simulink model "PenduloCarro2"  (R2017b)
settings: Solver=ode4  StartTime=0.0  StopTime=10.0  FixedStep=0.001  RelTol=1e-3
values from neighbouring files (symbols this model uses):
  g = 9.81    [PenduloInvertido.m]
  l = 0.5    [PenduloInvertido.m]
  m = 0.1    [PenduloInvertido.m]
undefined symbols (not defined in the file or in its folder): K, m1
settings Model: Creator=Benjamin Nicolas  LastModifiedBy=Benjamin Nicolas

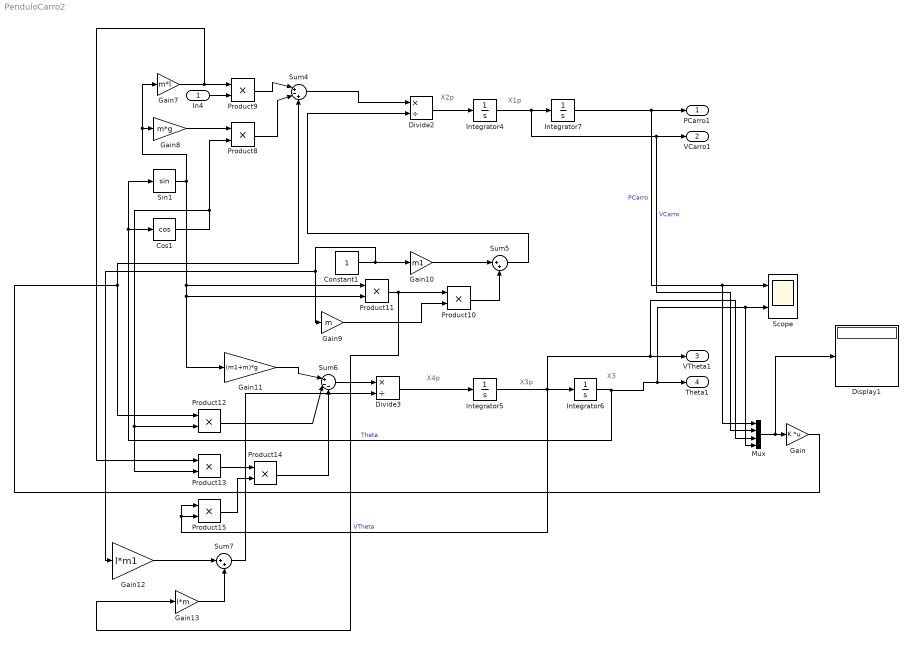
== system PenduloCarro2 ==
  note: X3
  note: X1p
  note: X2p
  note: X4p
  note: X3p
  In4 : Inport
  Constant1 : Constant
  Cos1 : Trigonometry  Operator=cos
  Display1 : Display
  Divide2 : Product  Inputs=*/
  Divide3 : Product  Inputs=*/
  Gain : Gain  Gain=K  Multiplication=Matrix(K*u)
  Gain10 : Gain  Gain=m1
  Gain11 : Gain  Gain=(m1+m)*g
  Gain12 : Gain  Gain=l*m1
  Gain13 : Gain  Gain=l*m
  Gain7 : Gain  Gain=m*l
  Gain8 : Gain  Gain=m*g
  Gain9 : Gain  Gain=m
  Integrator4 : Integrator
  Integrator5 : Integrator  InitialCondition=0.13
  Integrator6 : Integrator
  Integrator7 : Integrator
  Mux : Mux
  Product{8..15} (8 alike) : Product
  Scope : Scope  NumInputPorts=2
  Sin1 : Trigonometry
  Sum4 : Sum  Inputs=|+-+
  Sum5 : Sum  Inputs=|++
  Sum6 : Sum  Inputs=|+--
  Sum7 : Sum  Inputs=|++
  PCarro1 : Outport
  VCarro1 : Outport  Port=2
  VTheta1 : Outport  Port=3
  Theta1 : Outport  Port=4
  wires:
  Gain/1 -> Sum4/3, Product12/1
  Integrator7/1 -> Mux/1, Scope/1, PCarro1/1  "PCarro"
  Product8/1 -> Sum4/2
  Integrator4/1 -> Mux/2, VCarro1/1, Integrator7/1  "VCarro"
  Gain8/1 -> Product8/1
  Gain7/1 -> Product13/1, Product9/1
  Sum7/1 -> Divide3/2
  Product13/1 -> Product14/1
  Sum6/1 -> Divide3/1
  Gain10/1 -> Sum5/1
  Gain12/1 -> Sum7/1
  Gain13/1 -> Sum7/2
  Sum5/1 -> Divide2/2
  Gain11/1 -> Sum6/1
  Gain9/1 -> Product10/2
  Product14/1 -> Sum6/3
  Product9/1 -> Sum4/1
  In4/1 -> Product9/2
  Product12/1 -> Sum6/2
  Sin1/1 -> Gain11/1, Product11/2, Product11/1, Gain7/1, Gain8/1
  Cos1/1 -> Product12/2, Product13/2, Product8/2
  Product10/1 -> Sum5/2
  Constant1/1 -> Gain12/1, Gain9/1, Gain10/1
  Integrator5/1 -> Mux/3, VTheta1/1, Integrator6/1, Product15/2, Product15/1  "VTheta"
  Product15/1 -> Product14/2
  Integrator6/1 -> Mux/4, Scope/2, Theta1/1, Sin1/1, Cos1/1  "Theta"
  Product11/1 -> Gain13/1, Product10/1
  Sum4/1 -> Divide2/1
  Divide3/1 -> Integrator5/1
  Divide2/1 -> Integrator4/1
  Mux/1 -> Display1/1, Gain/1
